simulink library "sixDoFDynamicsEuler_ul"  (R2018b)
settings: Solver=VariableStepAuto  StartTime=0.0  StopTime=10.0  RelTol=1e-3
undefined symbols (not defined in the file): initAngRates, initAngVel, initEulAngs, initPos, initVel, J, J_added, Jinv, Jtot, M, M_added, Minv
libraries: vrlib x2, simulink x1, eulAng2RotMat_ul x1, eulDot x1
settings Model: Creator=mcobb  LastModifiedBy=asiddiq2

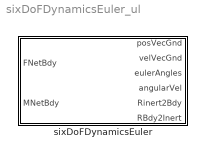
== system sixDoFDynamicsEuler_ul ==
  sixDoFDynamicsEuler : Subsystem  VariantControl=(default)  mask{M=M, M_added=M_added, J=J, J_added=J_added, initPos=initPos, initVel=initVel, initEulAngs=initEulAngs, initAngVel=initAngVel}
      mask prompts: M "Mass"; M_added "Added mass matrix"; J "Inertia matrix"; J_added "Added inertia matrix"; initPos "Initial position"; initVel "Initial velocity"; initEulAngs "Initial Euler Angles"; initAngVel "Initial Angular Velocity Vec"
      mask init:
      | sixDoFDynamics_init

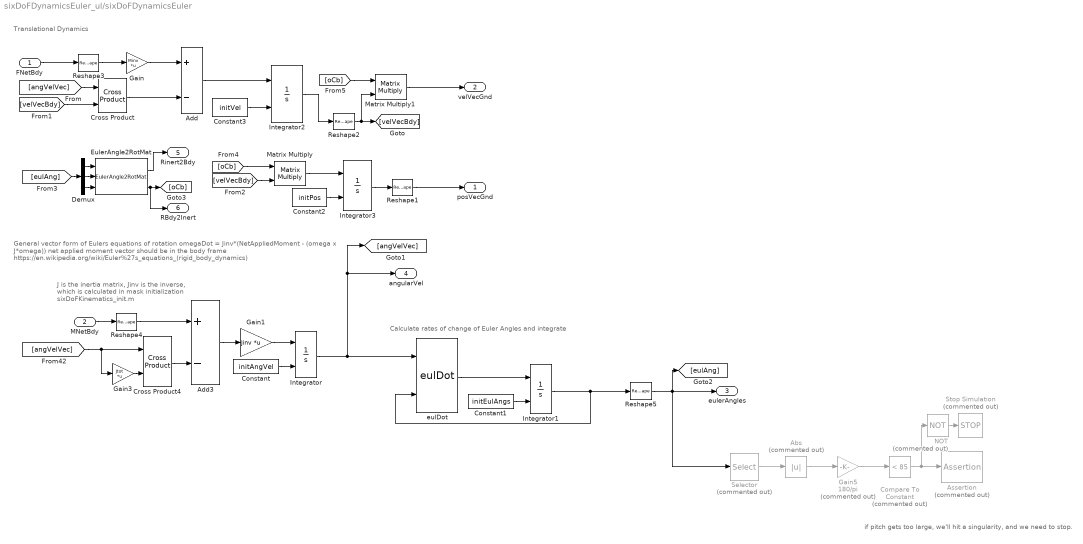
== system sixDoFDynamicsEuler_ul/sixDoFDynamicsEuler ==
  note: Translational Dynamics
  note: Calculate rates of change of Euler Angles and integrate
  note: General vector form of Eulers equations of rotation
      | omegaDot = Jinv*(NetAppliedMoment - (omega x J*omega))
      | net applied moment vector should be in the body frame
      | https://en.wikipedia.org/wiki/Euler%27s_equations_(rigid_body_dynamics)
  note: J is the inertia matrix, Jinv is the inverse,
      | which is calculated in mask initialization
      | sixDoFKinematics_init.m
  note: if pitch gets too large, we'll hit a singularity, and we need to stop.
  FNetBdy : Inport
  MNetBdy : Inport  Port=2
  Abs : Abs  Commented=on
  Add : Sum  Inputs=+-
  Add3 : Sum  Inputs=+-
  Assertion : Assertion  Commented=on  AssertionFailFcn="fprintf(2,\"Exiting because pitch exceeded 85 degrees.\\nThrowing Assertion Warning...\\n\")"  StopWhenAssertionFail=off
  Compare To Constant : simulink/Logic and Bit Operations/Compare To Constant  Commented=on  relop=<  const=85  OutDataTypeStr=boolean
  Constant : Constant  Value=initAngVel
  Constant1 : Constant  Value=initEulAngs
  Constant2 : Constant  Value=initPos
  Constant3 : Constant  Value=initVel
  Cross Product : vrlib/Utilities/Cross Product
      settings: SourceProductBaseCode=VR
  Cross Product4 : vrlib/Utilities/Cross Product
      settings: SourceProductBaseCode=VR
  Demux : Demux  Outputs=3
  EulerAngle2RotMat : eulAng2RotMat_ul/EulerAngle2RotMat  SystemSampleTime=-1
  Gain : Gain  Gain=Minv  Multiplication=Matrix(K*u)
  Gain1 : Gain  Gain=Jinv  Multiplication=Matrix(K*u)
  Gain3 : Gain  Gain=Jtot  Multiplication=Matrix(K*u)
  Gain5 : Gain  Commented=on  Gain=180/pi
  Integrator : Integrator  InitialConditionSource=external  InitialCondition=initAngRates
  Integrator1 : Integrator  InitialConditionSource=external  InitialCondition=initEulAngs
  Integrator2 : Integrator  InitialConditionSource=external  InitialCondition=initVel
  Integrator3 : Integrator  InitialConditionSource=external  InitialCondition=initPos
  Matrix Multiply : Product  Multiplication=Matrix(*)
  Matrix Multiply1 : Product  Multiplication=Matrix(*)
  NOT : Logic  Commented=on  Operator=NOT  IconShape=distinctive  AllPortsSameDT=off  OutDataTypeStr=boolean
  Reshape{1..5} (5 alike) : Reshape  OutputDimensionality=Column vector (2-D)
  Selector : Selector  Commented=on  InputPortWidth=3  IndexOptions=Index vector (dialog)  Indices=2  OutputSizes=1
  Stop Simulation : Stop  Commented=on
  eulDot : eulDot/eulDot  SystemSampleTime=-1
  posVecGnd : Outport
  velVecGnd : Outport  Port=2
  eulerAngles : Outport  Port=3
  angularVel : Outport  Port=4
  Rinert2Bdy : Outport  Port=5
  RBdy2Inert : Outport  Port=6
  wires:
  Reshape4/1 -> Add3/1
  NOT/1 -> Stop Simulation/1
  Gain/1 -> Add/1
  Compare To Constant/1 -> NOT/1, Assertion/1
  EulerAngle2RotMat/1 -> Rinert2Bdy/1
  [oCb] -> Matrix Multiply1/1
  Reshape1/1 -> posVecGnd/1
  Constant3/1 -> Integrator2/2
  Abs/1 -> Gain5/1
  Gain5/1 -> Compare To Constant/1
  Matrix Multiply1/1 -> velVecGnd/1
  [oCb] -> Matrix Multiply/1
  Selector/1 -> Abs/1
  Cross Product4/1 -> Add3/2
  Integrator1/1 -> eulDot/2, Reshape5/1
  Integrator/1 -> eulDot/1, angularVel/1, [angVelVec]
  MNetBdy/1 -> Reshape4/1
  Cross Product/1 -> Add/2
  Add/1 -> Integrator2/1
  Demux/3 -> EulerAngle2RotMat/3
  Demux/1 -> EulerAngle2RotMat/1
  [velVecBdy] -> Cross Product/2
  Matrix Multiply/1 -> Integrator3/1
  Add3/1 -> Gain1/1
  Reshape3/1 -> Gain/1
  [velVecBdy] -> Matrix Multiply/2
  Reshape5/1 -> Selector/1, eulerAngles/1, [eulAng]
  [angVelVec] -> Cross Product4/1, Gain3/1
  EulerAngle2RotMat/2 -> RBdy2Inert/1, [oCb]
  [eulAng] -> Demux/1
  Demux/2 -> EulerAngle2RotMat/2
  Constant2/1 -> Integrator3/2
  Integrator2/1 -> Reshape2/1
  FNetBdy/1 -> Reshape3/1
  eulDot/1 -> Integrator1/1
  [angVelVec] -> Cross Product/1
  Gain3/1 -> Cross Product4/2
  Reshape2/1 -> Matrix Multiply1/2, [velVecBdy]
  Constant/1 -> Integrator/2
  Constant1/1 -> Integrator1/2
  Gain1/1 -> Integrator/1
  Integrator3/1 -> Reshape1/1
